simulink model "dc_motor_model_with_chirp_sine"  (R2023a)
settings: Solver=VariableStepAuto  StartTime=0.0  StopTime=30  RelTol=1e-3
undefined symbols (not defined in the file or in its folder): a, K, Ke, T1
libraries: SignalEditorBlockLib x2, fuzblock x2, simulink x1, slpidlib x1
settings Model: Creator=Joe  LastModifiedBy=Joe

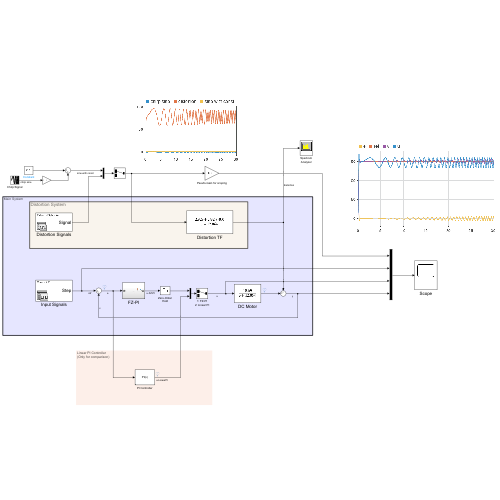
[thumbnail: Simulink's stored preview of the top-level diagram]
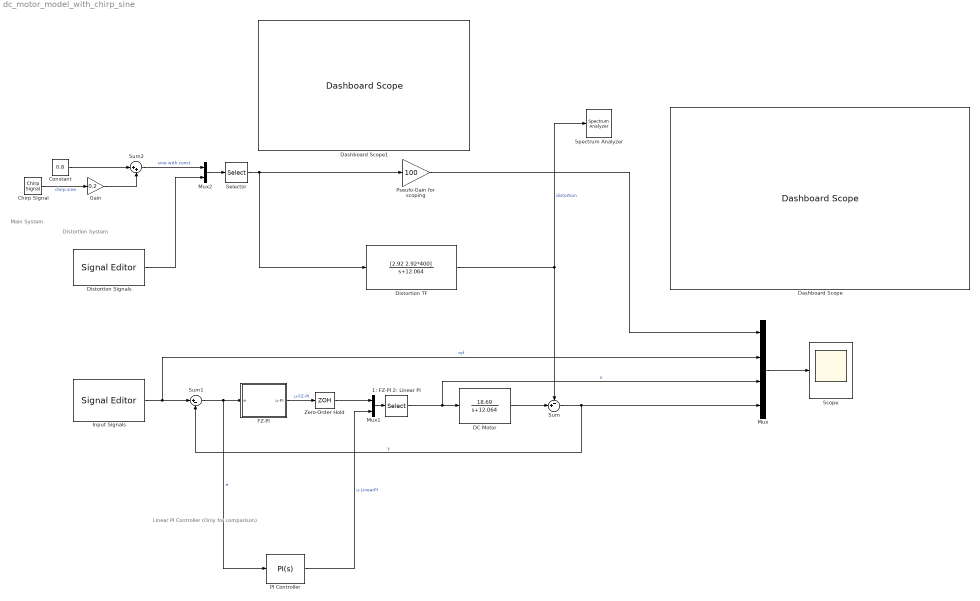
== system dc_motor_model_with_chirp_sine ==
  note: Distortion System
  note: Linear PI Controller
      | (Only for comparison)
  note: Main System
  1: FZ-PI 2: Linear PI : Selector  InputPortWidth=2  IndexOptions=Index vector (dialog)  Indices=1  OutputSizes=1
  Chirp Signal : simulink/Sources/Chirp Signal  f1=0.01  T=30  f2=2
  Constant : Constant  Value=0.8
  DC Motor : TransferFcn  Numerator=[18.69]  Denominator=[1 12.064]
  Dashboard Scope : DashboardScope  TimeSpan=30  Ymin=-20  Ymax=180
  Dashboard Scope1 : DashboardScope
  Distortion Signals : SignalEditorBlockLib/Signal Editor  FileName=external_distortion.mat  ActiveScenario=ExternalDistortion  ActiveSignal=Signal  IsBus=off  OutputBusObjectStr=Bus: BusObject  SampleTime=0  Interpolate=off  ZeroCross=off  OutputAfterFinalValue=Setting to zero  Unit=inherit  PreserveSignalName=on  ApplySigPropsToAllScenarios=on
  Distortion TF : TransferFcn  Numerator=[2.92 2.92*400]  Denominator=[1 12.064]
  FZ-PI : Subsystem
  Gain : Gain  Gain=0.2
  Input Signals : SignalEditorBlockLib/Signal Editor  FileName=input_scenarios.mat  ActiveScenario=Scenario3  ActiveSignal=Step  IsBus=off  OutputBusObjectStr=Bus: BusObject  SampleTime=0  Interpolate=off  ZeroCross=off  OutputAfterFinalValue=Setting to zero  Unit=V  PreserveSignalName=on  ApplySigPropsToAllScenarios=on
  Mux : Mux
  Mux1 : Mux  Inputs=2
  Mux2 : Mux  Inputs=2
  PI Controller : slpidlib/PID Controller  Controller=PI  Form=Parallel  TimeDomain=Continuous-time  UseExternalTs=off  SampleTime=-1  IntegratorMethod=Forward Euler  FilterMethod=Forward Euler  ControllerParametersSource=internal  P=1.25  I=10  UseKiTs=off  D=0  N=100  UseFilter=on  TunerSelectOption=Transfer Function Based (PID Tuner App)  InitialConditionSource=internal  InitialConditionForIntegrator=0  InitialConditionForFilter=0  DifferentiatorICPrevScaledInput=0  ExternalReset=none  TrackingMode=off  Kt=1  LimitOutput=off  SatLimitsSource=internal  UpperSaturationLimit=1  LowerSaturationLimit=-1  LinearizeAsGain=on  AntiWindupMode=clamping  Kb=1  LimitIntegrator=off  UpperIntegratorSaturationLimit=inf  LowerIntegratorSaturationLimit=-inf  RndMeth=Simplest  POutMin=[]  POutMax=[]  IOutMin=[]  IOutMax=[]  DOutMin=[]  DOutMax=[]  NOutMin=[]  NOutMax=[]  SumOutMin=[]  SumOutMax=[]  SaturationOutDataTypeStr=Inherit: Inherit via back propagation  SaturationOutMin=[]  SaturationOutMax=[]  PParamMin=[]  PParamMax=[]  IParamMin=[]  IParamMax=[]  DParamMin=[]  DParamMax=[]  NParamMin=[]  NParamMax=[]  KbParamMin=[]  KbParamMax=[]  KtParamMin=[]  KtParamMax=[]  KbOutMin=[]  KbOutMax=[]  KtOutMin=[]  KtOutMax=[]  IntegratorOutMin=[]  IntegratorOutMax=[]  FilterOutMin=[]  FilterOutMax=[]  SumI1OutMin=[]  SumI1OutMax=[]  SumI2OutMin=[]  SumI2OutMax=[]  SumI3OutMin=[]  SumI3OutMax=[]  SumI4OutMin=[]  SumI4OutMax=[]  SumDOutMin=[]  SumDOutMax=[]  DifferentiatorOutMin=[]  DifferentiatorOutMax=[]  FilterDiffOutCoefMin=[]  FilterDiffOutCoefMax=[]  ReciprocalOutMin=[]  ReciprocalOutMax=[]  SumDenOutMin=[]  SumDenOutMax=[]  SumNumOutMin=[]  SumNumOutMax=[]  DivideOutMin=[]  DivideOutMax=[]  UdiffTsProdOutMin=[]  UdiffTsProdOutMax=[]  NTsProdOutMin=[]  NTsProdOutMax=[]  UintegralTsProdOutMin=[]  UintegralTsProdOutMax=[]  UngainTsProdOutMin=[]  UngainTsProdOutMax=[]  ClampingZeroOutDataTypeStr=Inherit: Inherit via back propagation  ClampingZeroOutMin=[]  ClampingZeroOutMax=[]  FilterDenConstantOutDataTypeStr=Inherit: Inherit via back propagation  FilterDenConstantOutMin=[]  FilterDenConstantOutMax=[]  PCopyOutDataTypeStr=Inherit: Inherit via back propagation  PCopyOutMin=[]  PCopyOutMax=[]  NCopyOutDataTypeStr=Inherit: Inherit via back propagation  NCopyOutMin=[]  NCopyOutMax=[]  IntegratorContinuousStateAttributes=''  IntegratorStateMustResolveToSignalObject=off  IntegratorRTWStateStorageClass=Auto  FilterContinuousStateAttributes=''  FilterStateMustResolveToSignalObject=off  FilterRTWStateStorageClass=Auto  ParallelPVariant=InternalParameters  IdealPVariant=Disabled  IVariant=InternalParameters  DVariant=Disabled  IntegratorVariant=Continuous  SatVariant=Disabled  AWVariant=Passthrough  PCopyVariant=Disabled  TRVariant=Disabled  FdbkBlocksVariant=Forward  IdealPFdbkVariant=Disabled  SatFdbkVariant=Disabled  DerivativeFilterVariant=Disabled  NVariant=Disabled  NCopyVariant=Disabled_SignalSpec  FilterICVariant=Disabled  IntegratorICVariant=InternalICs  ExternalResetVariant=Disabled  TRSumVariant=Passthrough  SumFdbkVariant=Disabled  SumVariant=Sum_PI  TsampFilterVariant=InternalTs  TsampNgainVariant=Passthrough  TsampIntegralVariant=Disabled_SignalSpec  ExternalSaturationOutDataTypeStr=Inherit: Same as second input
      settings: LibrarySourceBlock=mcblib/Controls/Controllers/PI Controller
  Pseufo-Gain for scoping : Gain  Gain=100
  Scope : Scope
  Selector : Selector  InputPortWidth=2  IndexOptions=Index vector (dialog)  Indices=1  OutputSizes=1
  Spectrum Analyzer : SpectrumAnalyzer  WindowPosition=[273.000000,135.000000,996.000000,819.000000,]  ScopeFrameLocation=window  SampleRateSource=Property  SampleRate=44.1e3  PlotAsTwoSidedSpectrum=off  FrequencyScale=Log  FrequencySpan=Start and stop frequencies  StartFrequency=0.01  StopFrequency=5  YLimits=[-20,80]  ColorLimits=[-20 80]  ShowLegend=on  ExpandToolstrip=on  DefaultConfigurationName=spbscopes.SpectrumAnalyzerBlockCfg  IsFrequencyInputMode=0  FrequencyVectorPort=0  FrequencyVectorFromPort=0  FrequencyInputRBWPort=0  FrequencyInputRBWFromPort=0
  Sum : Sum  Inputs=-+|
  Sum1 : Sum  Inputs=|+-
  Sum2 : Sum  Inputs=|++
  Zero-Order Hold : ZeroOrderHold  SampleTime=0.01
  wires:
  DC Motor/1 -> Sum/2
  Distortion TF/1 -> Sum/1, Spectrum Analyzer/1  "distortion"
  Sum/1 -> Mux/4, Sum1/2  "y"
  Pseufo-Gain for scoping/1 -> Mux/1
  Sum1/1 -> PI Controller/1, FZ-PI/1(e)  "e"
  Input Signals/1 -> Mux/2, Sum1/1  "ref"
  Mux/1 -> Scope/1
  FZ-PI/1(u-PI) -> Zero-Order Hold/1  "u-FZ-PI"
  Zero-Order Hold/1 -> Mux1/1
  PI Controller/1 -> Mux1/2  "u-LinearPI"
  Mux1/1 -> 1: FZ-PI 2: Linear PI/1
  1: FZ-PI 2: Linear PI/1 -> Mux/3, DC Motor/1  "u"
  Selector/1 -> Distortion TF/1, Pseufo-Gain for scoping/1
  Mux2/1 -> Selector/1
  Distortion Signals/1 -> Mux2/2
  Sum2/1 -> Mux2/1  "sine with const"
  Constant/1 -> Sum2/1
  Gain/1 -> Sum2/2
  Chirp Signal/1 -> Gain/1  "chirp sine"

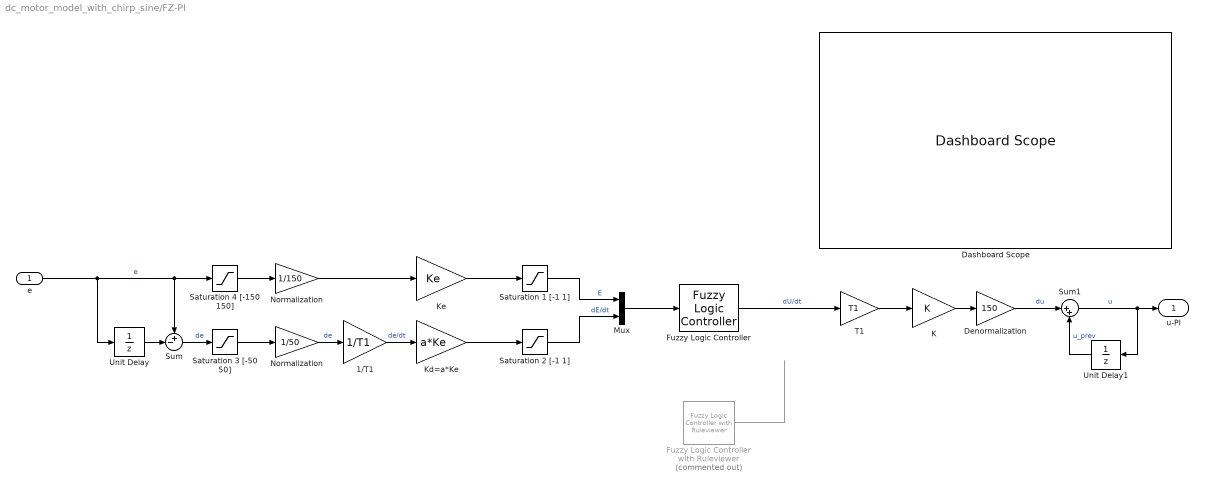
== system dc_motor_model_with_chirp_sine/FZ-PI ==
  e : Inport
  1/T1 : Gain  Gain=1/T1
  Dashboard Scope : DashboardScope
  Denormalization : Gain  Gain=150
  Fuzzy Logic Controller : fuzblock/Fuzzy Logic  Controller  FIS=flc_fis  OutputSampleNumber=101  DataType=double  FuzzifiedInputs=off  RuleFiringStrengths=off  RuleOutputs=off  AggregatedOutputs=off  SimulateUsing=Code generation  OutOfRangeInputValueMessage=warning  NoRuleFiredMessage=warning  EmptyOutputFuzzySetMessage=warning
  Fuzzy Logic Controller with Ruleviewer : fuzblock/Fuzzy Logic  Controller  with Ruleviewer  Commented=on  fismatrix=flc_fis  Ts=0.01
  K : Gain  Gain=K
  Kd=a*Ke : Gain  Gain=a*Ke
  Ke : Gain  Gain=Ke
  Mux : Mux  Inputs=2
  Normalization : Gain  Gain=1/50
  "Normalization " : Gain  Gain=1/150
  Saturation 1 [-1 1] : Saturate  UpperLimit=1  LowerLimit=-1
  Saturation 2 [-1 1] : Saturate  UpperLimit=1  LowerLimit=-1
  Saturation 3 [-50 50] : Saturate  UpperLimit=50  LowerLimit=-50
  Saturation 4 [-150 150] : Saturate  UpperLimit=150  LowerLimit=-150
  Sum : Sum  Inputs=+-|
  Sum1 : Sum  Inputs=|++
  T1 : Gain  Gain=T1
  Unit Delay : UnitDelay  SampleTime=-1  HasFrameUpgradeWarning=on
  Unit Delay1 : UnitDelay  SampleTime=-1  HasFrameUpgradeWarning=on
  u-PI : Outport  VectorParamsAs1DForOutWhenUnconnected=off
  wires:
  Saturation 1 [-1 1]/1 -> Mux/1  "E"
  Unit Delay1/1 -> Sum1/2  "u_prev"
  Denormalization/1 -> Sum1/1  "du"
  Unit Delay/1 -> Sum/2
  T1/1 -> K/1
  Saturation 2 [-1 1]/1 -> Mux/2  "dE/dt"
  Ke/1 -> Saturation 1 [-1 1]/1
  Sum1/1 -> Unit Delay1/1, u-PI/1  "u"
  K/1 -> Denormalization/1
  Mux/1 -> Fuzzy Logic Controller/1
  Sum/1 -> Saturation 3 [-50 50]/1  "de"
  e/1 -> Sum/1, Saturation 4 [-150 150]/1, Unit Delay/1  "e"
  Kd=a*Ke/1 -> Saturation 2 [-1 1]/1
  "Normalization "/1 -> Ke/1
  Saturation 3 [-50 50]/1 -> Normalization/1
  Normalization/1 -> 1/T1/1  "de"
  Saturation 4 [-150 150]/1 -> "Normalization "/1
  Fuzzy Logic Controller with Ruleviewer/1 -> ?
  Fuzzy Logic Controller/1 -> T1/1  "dU/dt"
  1/T1/1 -> Kd=a*Ke/1  "de/dt"
  ? -> Fuzzy Logic Controller with Ruleviewer/1
